simulink model "models"  (R2022a)
settings: Solver=VariableStepAuto  StartTime=0.0  StopTime=5  RelTol=1e-3
values from neighbouring files (symbols this model uses):
  k = 7    [task1.m]
  y0 = 1    [setconfig.m]
  y0dot1 = 0    [setconfig.m]
settings Model: Creator=Administrator  LastModifiedBy=Administrator

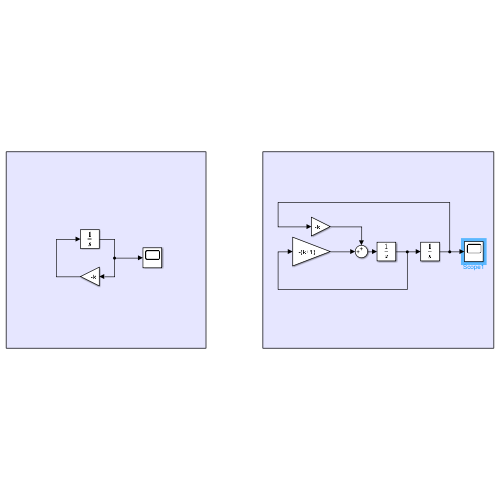
[thumbnail: Simulink's stored preview of the top-level diagram]
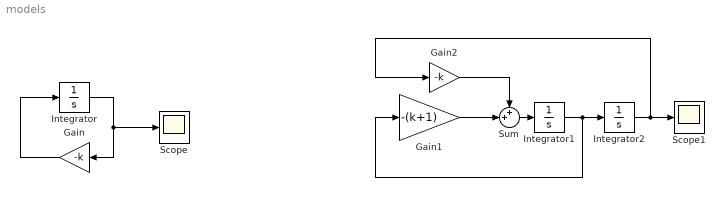
== system models ==
  Gain : Gain  Gain=-k
  Gain1 : Gain  Gain=-(k+1)
  Gain2 : Gain  Gain=-k
  Integrator : Integrator  InitialCondition=y0
  Integrator1 : Integrator  InitialCondition=y0dot1
  Integrator2 : Integrator  InitialCondition=y0
  Scope : Scope
  Scope1 : Scope
  Sum : Sum  Inputs=++|
  wires:
  Integrator/1 -> Gain/1, Scope/1
  Gain/1 -> Integrator/1
  Integrator1/1 -> Gain1/1, Integrator2/1
  Gain1/1 -> Sum/2
  Sum/1 -> Integrator1/1
  Gain2/1 -> Sum/1
  Integrator2/1 -> Scope1/1, Gain2/1
